simulink model "SF049A_LoaMgr"  (R2013b)
settings: Solver=FixedStepDiscrete  SolverMode=SingleTasking  StartTime=0.0  StopTime=1  FixedStep=0.002  RelTol=1e-3
values from neighbouring files (symbols this model uses):
  CURRMEASLOAMTGTNMASK_CNT_U08 = DataDict.Constant    [SF049A_LoaMgr_DataDict.m]
  IVTRLOAMTGTNMASK_CNT_U08 = DataDict.Constant    [SF049A_LoaMgr_DataDict.m]
  LOAMAXSLEW_ULSPERSEC_F32 = DataDict.Constant    [SF049A_LoaMgr_DataDict.m]
  LoaMgrCurrIvtrMtgtnRate = DataDict.Calibration    [SF049A_LoaMgr_DataDict.m]
  LoaMgrCurrIvtrMtgtnSca = DataDict.Calibration    [SF049A_LoaMgr_DataDict.m]
  LoaMgrCurrIvtrMtgtnScaZeroEna = DataDict.Calibration    [SF049A_LoaMgr_DataDict.m]
  LoaMgrCurrMeasIdptSig0Resp = DataDict.Calibration    [SF049A_LoaMgr_DataDict.m]
  LoaMgrCurrMeasIdptSig1Resp = DataDict.Calibration    [SF049A_LoaMgr_DataDict.m]
  LoaMgrCurrMeasIdptSig2Resp = DataDict.Calibration    [SF049A_LoaMgr_DataDict.m]
  LoaMgrCurrMeasIdptSigFltThd = DataDict.Calibration    [SF049A_LoaMgr_DataDict.m]
  LoaMgrCurrMeasMtgtnRate = DataDict.Calibration    [SF049A_LoaMgr_DataDict.m]
  LoaMgrCurrMeasMtgtnSca = DataDict.Calibration    [SF049A_LoaMgr_DataDict.m]
  LoaMgrCurrMeasMtgtnScaZeroEna = DataDict.Calibration    [SF049A_LoaMgr_DataDict.m]
  LoaMgrFadeOutStRate = DataDict.Calibration    [SF049A_LoaMgr_DataDict.m]
  LoaMgrHwTqIdptSig0NoTqLoaResp = DataDict.Calibration    [SF049A_LoaMgr_DataDict.m]
  LoaMgrHwTqIdptSig1NoTqLoaResp = DataDict.Calibration    [SF049A_LoaMgr_DataDict.m]
  LoaMgrHwTqIdptSig2Resp = DataDict.Calibration    [SF049A_LoaMgr_DataDict.m]
  LoaMgrHwTqIdptSig4Resp = DataDict.Calibration    [SF049A_LoaMgr_DataDict.m]
  LoaMgrHwTqIdptSigFltThd = DataDict.Calibration    [SF049A_LoaMgr_DataDict.m]
  LoaMgrHwTqLoaAvlResp = DataDict.Calibration    [SF049A_LoaMgr_DataDict.m]
  LoaMgrIvtrIdptSig0Resp = DataDict.Calibration    [SF049A_LoaMgr_DataDict.m]
  LoaMgrIvtrIdptSig1Resp = DataDict.Calibration    [SF049A_LoaMgr_DataDict.m]
  LoaMgrIvtrIdptSig2Resp = DataDict.Calibration    [SF049A_LoaMgr_DataDict.m]
  LoaMgrIvtrIdptSigFltThd = DataDict.Calibration    [SF049A_LoaMgr_DataDict.m]
  LoaMgrIvtrMtgtnRate = DataDict.Calibration    [SF049A_LoaMgr_DataDict.m]
  LoaMgrIvtrMtgtnSca = DataDict.Calibration    [SF049A_LoaMgr_DataDict.m]
  LoaMgrIvtrMtgtnScaZeroEna = DataDict.Calibration    [SF049A_LoaMgr_DataDict.m]
  LoaMgrLimdStRate = DataDict.Calibration    [SF049A_LoaMgr_DataDict.m]
  LoaMgrLimdStSca = DataDict.Calibration    [SF049A_LoaMgr_DataDict.m]
  LoaMgrMotAgAvlSnsrlsResp = DataDict.Calibration    [SF049A_LoaMgr_DataDict.m]
  LoaMgrMotAgIdptSig0NoSnsrlsResp = DataDict.Calibration    [SF049A_LoaMgr_DataDict.m]
  LoaMgrMotAgIdptSig1NoSnsrlsResp = DataDict.Calibration    [SF049A_LoaMgr_DataDict.m]
  LoaMgrMotAgIdptSig2Resp = DataDict.Calibration    [SF049A_LoaMgr_DataDict.m]
  LoaMgrMotAgIdptSig3Resp = DataDict.Calibration    [SF049A_LoaMgr_DataDict.m]
  LoaMgrMotAgIdptSigFltThd = DataDict.Calibration    [SF049A_LoaMgr_DataDict.m]
  LoaMgrMotAgMtgtnRate = DataDict.Calibration    [SF049A_LoaMgr_DataDict.m]
  LoaMgrMotAgMtgtnSca = DataDict.Calibration    [SF049A_LoaMgr_DataDict.m]
  LoaMgrMotAgMtgtnScaZeroEna = DataDict.Calibration    [SF049A_LoaMgr_DataDict.m]
  LOASCAONE_ULS_F32 = DataDict.Constant    [SF049A_LoaMgr_DataDict.m]
  LOASCAZERO_ULS_F32 = DataDict.Constant    [SF049A_LoaMgr_DataDict.m]
  LOASTIMDTSHTDWN_CNT_U08 = DataDict.Constant    [SF049A_LoaMgr_DataDict.m]
  LOASTNORM_CNT_U08 = DataDict.Constant    [SF049A_LoaMgr_DataDict.m]
  LOASTSWMTGTN_CNT_U08 = DataDict.Constant    [SF049A_LoaMgr_DataDict.m]
  MAXCURRMEASIDPTSIGALLWD_CNT_U08 = DataDict.Constant    [SF049A_LoaMgr_DataDict.m]
  MAXHWTQIDPTSIGALLWD_CNT_U08 = DataDict.Constant    [SF049A_LoaMgr_DataDict.m]
  MAXIVTRIDPTSIGALLWD_CNT_U08 = DataDict.Constant    [SF049A_LoaMgr_DataDict.m]
  MAXMOTAGMECLIDPTSIGALLWD_CNT_U08 = DataDict.Constant    [SF049A_LoaMgr_DataDict.m]
  NODEBSTEP_CNT_U16 = DataDict.Constant    [SF049A_LoaMgr_DataDict.m]
undefined symbols (not defined in the file or in its folder): LoaSt1, NtcNr1, NtcSts1, SigQlfr1
libraries: simulink x43, NxtrMin x4, NxtrMax x4, NxtrLim x2
(part 3 of 8)

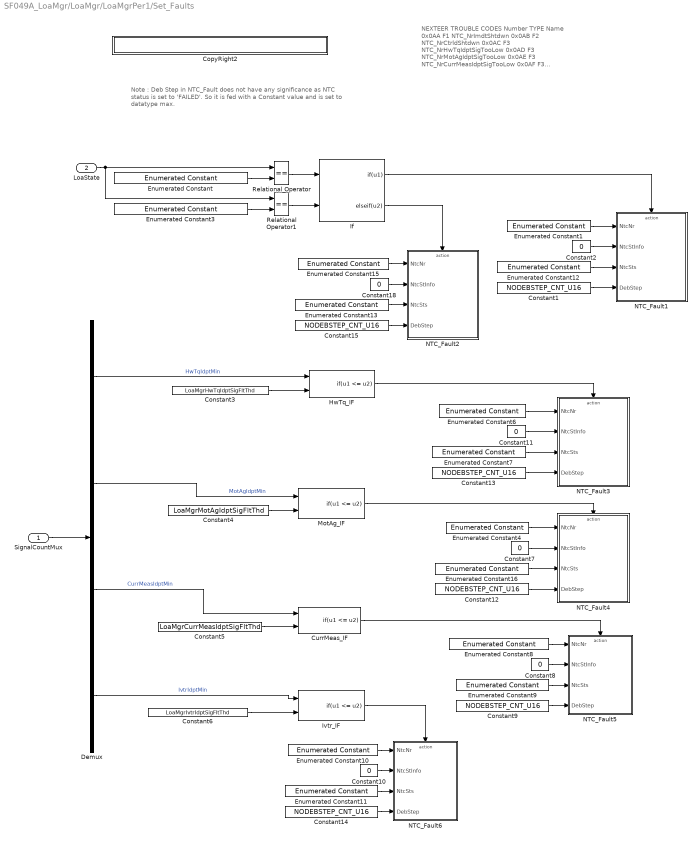
== system SF049A_LoaMgr/LoaMgr/LoaMgrPer1/Set_Faults ==
  note: Note : Deb Step in NTC_Fault does not have any significance as
      | NTC status is set to 'FAILED'. So it is fed with a Constant value and
      | is set to datatype max.
  note: NEXTEER TROUBLE CODES
      | Number  TYPE   Name
      |  0x0AA      F1      NTC_NrImdtShtdwn
      |  0x0AB      F2      NTC_NrCtrldShtdwn
      |  0x0AC      F3      NTC_NrHwTqIdptSigTooLow
      |  0x0AD      F3      NTC_NrMotAgIdptSigTooLow
      |  0x0AE      F3      NTC_NrCurrMeasIdptSigTooLow
      |  0x0AF      F3      NTC_NrIvtrIdptSigTooLow
  SignalCountMux : Inport
  LoaState : Inport  RequirementInfo="{'linktype_rmi_doors' '0000bab3 (/E-STEER Core/SubSystem Specifications/Application Functions/SF049A Loss of Assist Manager)' '#SF049A_115' 'true' 'REQ:  SF049A_115' '' ; 'linktype_rmi_doors' '0000bab3 (/E-STEER Core/SubSystem Specifications/Application Functions/SF049A Loss of Assist Manager)' '#SF049A_118' 'true' 'REQ:  SF049A_118' '' } %GIDa_4967d76f_74bb_495b_9f1d_be295f669af9"  Port=2
  Constant{1,9,12..15} (6 alike) : Constant  Value=NODEBSTEP_CNT_U16
  Constant{2,7..8,10..11,18} (6 alike) : Constant  Value=0
  Constant3 : Constant  RequirementInfo="{'linktype_rmi_doors' '0000bab3 (/E-STEER Core/SubSystem Specifications/Application Functions/SF049A Loss of Assist Manager)' '#SF049A_127' 'true' 'REQ:  SF049A_127' '' } %GIDa_3c5e0169_e7e2_4269_822a_0506f737a0d4"  Value=LoaMgrHwTqIdptSigFltThd  OutDataTypeStr=uint8
  Constant4 : Constant  RequirementInfo="{'linktype_rmi_doors' '0000bab3 (/E-STEER Core/SubSystem Specifications/Application Functions/SF049A Loss of Assist Manager)' '#SF049A_136' 'true' 'REQ:  SF049A_136' '' } %GIDa_abce65b2_de1a_4f6f_b7d5_5b7546b3af4d"  Value=LoaMgrMotAgIdptSigFltThd  OutDataTypeStr=uint8
  Constant5 : Constant  RequirementInfo="{'linktype_rmi_doors' '0000bab3 (/E-STEER Core/SubSystem Specifications/Application Functions/SF049A Loss of Assist Manager)' '#SF049A_145' 'true' 'REQ:  SF049A_145' '' } %GIDa_8ca978df_ec13_4868_a0a0_36ae85151f3c"  Value=LoaMgrCurrMeasIdptSigFltThd  OutDataTypeStr=uint8
  Constant6 : Constant  RequirementInfo="{'linktype_rmi_doors' '0000bab3 (/E-STEER Core/SubSystem Specifications/Application Functions/SF049A Loss of Assist Manager)' '#SF049A_154' 'true' 'REQ:  SF049A_154' '' } %GIDa_e4e38833_0b1e_42a6_94e4_589df1509d92"  Value=LoaMgrIvtrIdptSigFltThd  OutDataTypeStr=uint8
  CopyRight2 : Subsystem  Description=|  mask(Copyright Information){none=on}
      | Copyright info block.                                               
      |                                                                     
      | Place copyright information at the top of every subsystem in design.
      mask prompts: none "No parameters"
      mask help: Place copyright information at the top of every subsystem in design.
      mask Display:
      | NxtrConf = 'Nexteer Confidential';
      | 
      | sys = bdroot; %handle for the current model ("system")
      | first = get_param(sys,'Created');
      | first = first(end-3:end);  %year is last four digits
      | 
      | last = get_param(sys,'LastModifiedDate');
      | if isempty(last)
      |     last = datestr(now,'yyyy');
      | else
      |     last = last(end-3:end);
      | end
      | 
      | if strcmp(first,last)
      |     fprintf('%s -- Copyright %s Nexteer',NxtrConf,first)
      | else
      |     fprintf('%s -- %s%s- %s Nexteer',NxtrConf,char(169),first,last)
      | end
  CurrMeas_IF : If  RequirementInfo="{'linktype_rmi_doors' '0000bab3 (/E-STEER Core/SubSystem Specifications/Application Functions/SF049A Loss of Assist Manager)' '#SF049A_145' 'true' 'REQ:  SF049A_145' '' } %GIDa_23c69e12_f1ab_48c3_a465_95305b9e4132"  NumInputs=2  IfExpression=u1 <= u2  ShowElse=off
  Demux : Demux
  Enumerated Constant1 : simulink/Sources/Enumerated Constant  OutDataTypeStr=Enum: NtcNr1  Value=NtcNr1.NTCNR_0X0AA  SampleTime=inf
  Enumerated Constant10 : simulink/Sources/Enumerated Constant  OutDataTypeStr=Enum: NtcNr1  Value=NtcNr1.NTCNR_0X0AF  SampleTime=inf
  Enumerated Constant{7,9,11..13,16} (6 alike) : simulink/Sources/Enumerated Constant  OutDataTypeStr=Enum: NtcSts1  Value=NtcSts1.NTCSTS_FAILD  SampleTime=inf
  Enumerated Constant15 : simulink/Sources/Enumerated Constant  OutDataTypeStr=Enum: NtcNr1  Value=NtcNr1.NTCNR_0X0AB  SampleTime=inf
  Enumerated Constant4 : simulink/Sources/Enumerated Constant  OutDataTypeStr=Enum: NtcNr1  Value=NtcNr1.NTCNR_0X0AD  SampleTime=inf
  Enumerated Constant6 : simulink/Sources/Enumerated Constant  OutDataTypeStr=Enum: NtcNr1  Value=NtcNr1.NTCNR_0X0AC  SampleTime=inf
  Enumerated Constant8 : simulink/Sources/Enumerated Constant  OutDataTypeStr=Enum: NtcNr1  Value=NtcNr1.NTCNR_0X0AE  SampleTime=inf
  Enumerated Constant : simulink/Sources/Enumerated Constant  RequirementInfo="{'linktype_rmi_doors' '0000bab3 (/E-STEER Core/SubSystem Specifications/Application Functions/SF049A Loss of Assist Manager)' '#SF049A_115' 'true' 'REQ:  SF049A_115' '' } %GIDa_7720fc81_938d_420c_9ced_1233460611ba"  OutDataTypeStr=Enum: LoaSt1  Value=LoaSt1.LOAST_IMDTSHTDWNREQD  SampleTime=inf
  Enumerated Constant3 : simulink/Sources/Enumerated Constant  RequirementInfo="{'linktype_rmi_doors' '0000bab3 (/E-STEER Core/SubSystem Specifications/Application Functions/SF049A Loss of Assist Manager)' '#SF049A_118' 'true' 'REQ:  SF049A_118' '' } %GIDa_0b8c704e_8242_4dec_ad1d_b890924ca18f"  OutDataTypeStr=Enum: LoaSt1  Value=LoaSt1.LOAST_CTRLDSHTDWNREQD  SampleTime=inf
  HwTq_IF : If  RequirementInfo="{'linktype_rmi_doors' '0000bab3 (/E-STEER Core/SubSystem Specifications/Application Functions/SF049A Loss of Assist Manager)' '#SF049A_127' 'true' 'REQ:  SF049A_127' '' } %GIDa_c1a54aec_df59_476e_b8a2_fe90d0d01382"  NumInputs=2  IfExpression=u1 <= u2  ShowElse=off
  If : If  RequirementInfo="{'linktype_rmi_doors' '0000bab3 (/E-STEER Core/SubSystem Specifications/Application Functions/SF049A Loss of Assist Manager)' '#SF049A_115' 'true' 'REQ:  SF049A_115' '' ; 'linktype_rmi_doors' '0000bab3 (/E-STEER Core/SubSystem Specifications/Application Functions/SF049A Loss of Assist Manager)' '#SF049A_118' 'true' 'REQ:  SF049A_118' '' } %GIDa_2ae57359_ddcb_46c2_bc65_be72e5cb3771"  NumInputs=2  IfExpression=u1  ElseIfExpressions=u2  ShowElse=off
  Ivtr_IF : If  RequirementInfo="{'linktype_rmi_doors' '0000bab3 (/E-STEER Core/SubSystem Specifications/Application Functions/SF049A Loss of Assist Manager)' '#SF049A_154' 'true' 'REQ:  SF049A_154' '' } %GIDa_9e953e66_734a_4534_a97e_ce62b3d493b7"  NumInputs=2  IfExpression=u1 <= u2  ShowElse=off
  MotAg_IF : If  RequirementInfo="{'linktype_rmi_doors' '0000bab3 (/E-STEER Core/SubSystem Specifications/Application Functions/SF049A Loss of Assist Manager)' '#SF049A_136' 'true' 'REQ:  SF049A_136' '' } %GIDa_2fb2f3b7_b2e9_48d1_9bc3_88796399833b"  NumInputs=2  IfExpression=u1 <= u2  ShowElse=off
  NTC_Fault1 : Subsystem  mask(SetNTC){}
      mask help: SetNTC library block
  NTC_Fault2 : Subsystem  mask(SetNTC){}
      mask help: SetNTC library block
  NTC_Fault3 : Subsystem  mask(SetNTC){}
      mask help: SetNTC library block
  NTC_Fault4 : Subsystem  mask(SetNTC){}
      mask help: SetNTC library block
  NTC_Fault5 : Subsystem  mask(SetNTC){}
      mask help: SetNTC library block
  NTC_Fault6 : Subsystem  mask(SetNTC){}
      mask help: SetNTC library block
  Relational Operator : RelationalOperator  RequirementInfo="{'linktype_rmi_doors' '0000bab3 (/E-STEER Core/SubSystem Specifications/Application Functions/SF049A Loss of Assist Manager)' '#SF049A_115' 'true' 'REQ:  SF049A_115' '' } %GIDa_f05a48eb_4c6a_4aaa_9a59_9f6400fec108"  Operator===  OutDataTypeStr=boolean
  Relational Operator1 : RelationalOperator  RequirementInfo="{'linktype_rmi_doors' '0000bab3 (/E-STEER Core/SubSystem Specifications/Application Functions/SF049A Loss of Assist Manager)' '#SF049A_118' 'true' 'REQ:  SF049A_118' '' } %GIDa_4de44a16_c7b2_4a4a_90aa_5030e7b317ef"  Operator===  OutDataTypeStr=boolean
  wires:
  If/2 -> NTC_Fault2/Action
  If/1 -> NTC_Fault1/Action
  Enumerated Constant/1 -> Relational Operator/2
  Enumerated Constant3/1 -> Relational Operator1/2
  LoaState/1 -> Relational Operator/1, Relational Operator1/1
  Relational Operator1/1 -> If/2
  Relational Operator/1 -> If/1
  SignalCountMux/1 -> Demux/1
  Constant3/1 -> HwTq_IF/2
  Demux/1 -> HwTq_IF/1  "HwTqIdptMin"
  Constant4/1 -> MotAg_IF/2
  Demux/2 -> MotAg_IF/1  "MotAgIdptMin"
  Constant5/1 -> CurrMeas_IF/2
  Demux/3 -> CurrMeas_IF/1  "CurrMeasIdptMin"
  Constant6/1 -> Ivtr_IF/2
  Demux/4 -> Ivtr_IF/1  "IvtrIdptMin"
  HwTq_IF/1 -> NTC_Fault3/Action
  MotAg_IF/1 -> NTC_Fault4/Action
  Enumerated Constant8/1 -> NTC_Fault5/1(NtcNr)
  Constant8/1 -> NTC_Fault5/2(NtcStInfo)
  Enumerated Constant9/1 -> NTC_Fault5/3(NtcSts)
  Constant9/1 -> NTC_Fault5/4(DebStep)
  CurrMeas_IF/1 -> NTC_Fault5/Action
  Enumerated Constant10/1 -> NTC_Fault6/1(NtcNr)
  Constant10/1 -> NTC_Fault6/2(NtcStInfo)
  Enumerated Constant11/1 -> NTC_Fault6/3(NtcSts)
  Constant14/1 -> NTC_Fault6/4(DebStep)
  Ivtr_IF/1 -> NTC_Fault6/Action
  Constant15/1 -> NTC_Fault2/4(DebStep)
  Enumerated Constant13/1 -> NTC_Fault2/3(NtcSts)
  Constant18/1 -> NTC_Fault2/2(NtcStInfo)
  Enumerated Constant15/1 -> NTC_Fault2/1(NtcNr)
  Enumerated Constant1/1 -> NTC_Fault1/1(NtcNr)
  Constant2/1 -> NTC_Fault1/2(NtcStInfo)
  Enumerated Constant12/1 -> NTC_Fault1/3(NtcSts)
  Constant1/1 -> NTC_Fault1/4(DebStep)
  Enumerated Constant4/1 -> NTC_Fault4/1(NtcNr)
  Constant7/1 -> NTC_Fault4/2(NtcStInfo)
  Enumerated Constant16/1 -> NTC_Fault4/3(NtcSts)
  Constant12/1 -> NTC_Fault4/4(DebStep)
  Enumerated Constant6/1 -> NTC_Fault3/1(NtcNr)
  Constant11/1 -> NTC_Fault3/2(NtcStInfo)
  Enumerated Constant7/1 -> NTC_Fault3/3(NtcSts)
  Constant13/1 -> NTC_Fault3/4(DebStep)

== system SF049A_LoaMgr/LoaMgr/LoaMgrPer1/else ==
  In1 : Inport
  Action Port : ActionPort  ActionType=else
  Out1 : Outport
  wires:
  In1/1 -> Out1/1

== system SF049A_LoaMgr/LoaMgr/LoaMgrPer1/if ==
  Action Port : ActionPort  ActionType=then
  Constant : Constant  OutDataTypeStr=Inherit: Inherit via back propagation
  Out1 : Outport
  wires:
  Constant/1 -> Out1/1

== system SF049A_LoaMgr/ISO Fault Debounce/DiagMgr/NTCSTS_PREFAILD/CopyRight2 ==

== system SF049A_LoaMgr/ISO Fault Debounce/DiagMgr/NTCSTS_PREFAILD/If Action Subsystem ==
  DS : Inport
  Qlf : Inport  Port=2
  Action Port : ActionPort  ActionType=then
  EAo : Outport
  Qlfo : Outport  Port=2
  wires:
  Qlf/1 -> Qlfo/1
  DS/1 -> EAo/1

== system SF049A_LoaMgr/ISO Fault Debounce/DiagMgr/NTCSTS_PREFAILD/If Action Subsystem1 ==
  DS : Inport
  EA : Inport  Port=2
  Qlf : Inport  Port=3
  TS : Inport  Port=4
  Action Port : ActionPort  ActionType=else
  CopyRight2 : Subsystem  Description=|  mask(Copyright Information){none=on}
      | Copyright info block.                                               
      |                                                                     
      | Place copyright information at the top of every subsystem in design.
      mask prompts: none "No parameters"
      mask help: Place copyright information at the top of every subsystem in design.
      mask Display:
      | NxtrConf = 'Nexteer Confidential';
      | 
      | sys = bdroot; %handle for the current model ("system")
      | first = get_param(sys,'Created');
      | first = first(end-3:end);  %year is last four digits
      | 
      | last = get_param(sys,'LastModifiedDate');
      | if isempty(last)
      |     last = datestr(now,'yyyy');
      | else
      |     last = last(end-3:end);
      | end
      | 
      | if strcmp(first,last)
      |     fprintf('%s -- Copyright %s Nexteer',NxtrConf,first)
      | else
      |     fprintf('%s -- %s%s- %s Nexteer',NxtrConf,char(169),first,last)
      | end
  If : If  NumInputs=2  IfExpression=u1 < u2
  If Action Subsystem : Subsystem  TreatAsAtomicUnit=on
  If Action Subsystem1 : Subsystem  TreatAsAtomicUnit=on
  Merge : Merge
  Merge1 : Merge
  QFFailed : Constant  Value=SigQlfr1.SIGQLFR_FAILD  OutDataTypeStr=Enum: SigQlfr1
  Sum : Sum  Inputs=|++
  EAo : Outport
  Qlfo : Outport  Port=2
  wires:
  DS/1 -> Sum/1
  EA/1 -> Sum/2
  Sum/1 -> If Action Subsystem/1(EA), If/1
  TS/1 -> If Action Subsystem1/1(EA), If/2
  If/2 -> If Action Subsystem1/Action
  If/1 -> If Action Subsystem/Action
  Qlf/1 -> If Action Subsystem/2(Qlf)
  QFFailed/1 -> If Action Subsystem1/2(Qlf)
  Merge1/1 -> Qlfo/1
  Merge/1 -> EAo/1
  If Action Subsystem1/1(EAo) -> Merge/1
  If Action Subsystem/1(EAo) -> Merge/2
  If Action Subsystem1/2(Qlfo) -> Merge1/1
  If Action Subsystem/2(Qlfo) -> Merge1/2

== system SF049A_LoaMgr/ISO Fault Debounce/DiagMgr/NTCSTS_PREPASSD/CopyRight2 ==

== system SF049A_LoaMgr/ISO Fault Debounce/DiagMgr/NTCSTS_PREPASSD/If Action Subsystem ==
  In1 : Inport
  In2 : Inport  Port=2
  Action Port : ActionPort  ActionType=then
  Out1 : Outport
  Out2 : Outport  Port=2
  wires:
  In1/1 -> Out1/1
  In2/1 -> Out2/1

== system SF049A_LoaMgr/ISO Fault Debounce/DiagMgr/NTCSTS_PREPASSD/If Action Subsystem1 ==
  In1 : Inport
  In2 : Inport  Port=2
  Action Port : ActionPort  ActionType=else
  Out1 : Outport
  Out2 : Outport  Port=2
  wires:
  In1/1 -> Out1/1
  In2/1 -> Out2/1

== system SF049A_LoaMgr/LoaMgr/LoaMgrInit1/NTC_Fault1/SetNtcSts ==
  NtcNr : Inport
  NtcStInfo : Inport  Port=2
  NtcSts : Inport  Port=3
  DebStep : Inport  Port=4
  CopyRight2 : Subsystem  Description=|  mask(Copyright Information){none=on}
      | Copyright info block.                                               
      |                                                                     
      | Place copyright information at the top of every subsystem in design.
      mask prompts: none "No parameters"
      mask help: Place copyright information at the top of every subsystem in design.
      mask Display:
      | NxtrConf = 'Nexteer Confidential';
      | 
      | sys = bdroot; %handle for the current model ("system")
      | first = get_param(sys,'Created');
      | first = first(end-3:end);  %year is last four digits
      | 
      | last = get_param(sys,'LastModifiedDate');
      | if isempty(last)
      |     last = datestr(now,'yyyy');
      | else
      |     last = last(end-3:end);
      | end
      | 
      | if strcmp(first,last)
      |     fprintf('%s -- Copyright %s Nexteer',NxtrConf,first)
      | else
      |     fprintf('%s -- %s%s- %s Nexteer',NxtrConf,char(169),first,last)
      | end
  Data Store Write1 : DataStoreWrite  DataStoreName=DebStep
  Data Store Write3 : DataStoreWrite  DataStoreName=Fault1_Status
  Terminator : Terminator
  Terminator1 : Terminator
  wires:
  NtcStInfo/1 -> Terminator1/1
  NtcNr/1 -> Terminator/1
  NtcSts/1 -> Data Store Write3/1
  DebStep/1 -> Data Store Write1/1

== system SF049A_LoaMgr/LoaMgr/LoaMgrInit1/NTC_Fault2/SetNtcSts ==
  NtcNr : Inport
  NtcStInfo : Inport  Port=2
  NtcSts : Inport  Port=3
  DebStep : Inport  Port=4
  CopyRight2 : Subsystem  Description=|  mask(Copyright Information){none=on}
      | Copyright info block.                                               
      |                                                                     
      | Place copyright information at the top of every subsystem in design.
      mask prompts: none "No parameters"
      mask help: Place copyright information at the top of every subsystem in design.
      mask Display:
      | NxtrConf = 'Nexteer Confidential';
      | 
      | sys = bdroot; %handle for the current model ("system")
      | first = get_param(sys,'Created');
      | first = first(end-3:end);  %year is last four digits
      | 
      | last = get_param(sys,'LastModifiedDate');
      | if isempty(last)
      |     last = datestr(now,'yyyy');
      | else
      |     last = last(end-3:end);
      | end
      | 
      | if strcmp(first,last)
      |     fprintf('%s -- Copyright %s Nexteer',NxtrConf,first)
      | else
      |     fprintf('%s -- %s%s- %s Nexteer',NxtrConf,char(169),first,last)
      | end
  Data Store Write1 : DataStoreWrite  DataStoreName=DebStep
  Data Store Write3 : DataStoreWrite  DataStoreName=Fault2_Status
  Terminator : Terminator
  Terminator1 : Terminator
  wires:
  DebStep/1 -> Data Store Write1/1
  NtcSts/1 -> Data Store Write3/1
  NtcNr/1 -> Terminator/1
  NtcStInfo/1 -> Terminator1/1

== system SF049A_LoaMgr/LoaMgr/LoaMgrInit1/NTC_Fault3/SetNtcSts ==
  NtcNr : Inport
  NtcStInfo : Inport  Port=2
  NtcSts : Inport  Port=3
  DebStep : Inport  Port=4
  CopyRight2 : Subsystem  Description=|  mask(Copyright Information){none=on}
      | Copyright info block.                                               
      |                                                                     
      | Place copyright information at the top of every subsystem in design.
      mask prompts: none "No parameters"
      mask help: Place copyright information at the top of every subsystem in design.
      mask Display:
      | NxtrConf = 'Nexteer Confidential';
      | 
      | sys = bdroot; %handle for the current model ("system")
      | first = get_param(sys,'Created');
      | first = first(end-3:end);  %year is last four digits
      | 
      | last = get_param(sys,'LastModifiedDate');
      | if isempty(last)
      |     last = datestr(now,'yyyy');
      | else
      |     last = last(end-3:end);
      | end
      | 
      | if strcmp(first,last)
      |     fprintf('%s -- Copyright %s Nexteer',NxtrConf,first)
      | else
      |     fprintf('%s -- %s%s- %s Nexteer',NxtrConf,char(169),first,last)
      | end
  Data Store Write1 : DataStoreWrite  DataStoreName=DebStep
  Data Store Write3 : DataStoreWrite  DataStoreName=Fault3_Status
  Terminator : Terminator
  Terminator1 : Terminator
  wires:
  DebStep/1 -> Data Store Write1/1
  NtcSts/1 -> Data Store Write3/1
  NtcNr/1 -> Terminator/1
  NtcStInfo/1 -> Terminator1/1

== system SF049A_LoaMgr/LoaMgr/LoaMgrInit1/NTC_Fault4/SetNtcSts ==
  NtcNr : Inport
  NtcStInfo : Inport  Port=2
  NtcSts : Inport  Port=3
  DebStep : Inport  Port=4
  CopyRight2 : Subsystem  Description=|  mask(Copyright Information){none=on}
      | Copyright info block.                                               
      |                                                                     
      | Place copyright information at the top of every subsystem in design.
      mask prompts: none "No parameters"
      mask help: Place copyright information at the top of every subsystem in design.
      mask Display:
      | NxtrConf = 'Nexteer Confidential';
      | 
      | sys = bdroot; %handle for the current model ("system")
      | first = get_param(sys,'Created');
      | first = first(end-3:end);  %year is last four digits
      | 
      | last = get_param(sys,'LastModifiedDate');
      | if isempty(last)
      |     last = datestr(now,'yyyy');
      | else
      |     last = last(end-3:end);
      | end
      | 
      | if strcmp(first,last)
      |     fprintf('%s -- Copyright %s Nexteer',NxtrConf,first)
      | else
      |     fprintf('%s -- %s%s- %s Nexteer',NxtrConf,char(169),first,last)
      | end
  Data Store Write1 : DataStoreWrite  DataStoreName=DebStep
  Data Store Write3 : DataStoreWrite  DataStoreName=Fault4_Status
  Terminator : Terminator
  Terminator1 : Terminator
  wires:
  NtcStInfo/1 -> Terminator1/1
  NtcNr/1 -> Terminator/1
  NtcSts/1 -> Data Store Write3/1
  DebStep/1 -> Data Store Write1/1

== system SF049A_LoaMgr/LoaMgr/LoaMgrInit1/NTC_Fault5/SetNtcSts ==
  NtcNr : Inport
  NtcStInfo : Inport  Port=2
  NtcSts : Inport  Port=3
  DebStep : Inport  Port=4
  CopyRight2 : Subsystem  Description=|  mask(Copyright Information){none=on}
      | Copyright info block.                                               
      |                                                                     
      | Place copyright information at the top of every subsystem in design.
      mask prompts: none "No parameters"
      mask help: Place copyright information at the top of every subsystem in design.
      mask Display:
      | NxtrConf = 'Nexteer Confidential';
      | 
      | sys = bdroot; %handle for the current model ("system")
      | first = get_param(sys,'Created');
      | first = first(end-3:end);  %year is last four digits
      | 
      | last = get_param(sys,'LastModifiedDate');
      | if isempty(last)
      |     last = datestr(now,'yyyy');
      | else
      |     last = last(end-3:end);
      | end
      | 
      | if strcmp(first,last)
      |     fprintf('%s -- Copyright %s Nexteer',NxtrConf,first)
      | else
      |     fprintf('%s -- %s%s- %s Nexteer',NxtrConf,char(169),first,last)
      | end
  Data Store Write1 : DataStoreWrite  DataStoreName=DebStep
  Data Store Write3 : DataStoreWrite  DataStoreName=Fault5_Status
  Terminator : Terminator
  Terminator1 : Terminator
  wires:
  DebStep/1 -> Data Store Write1/1
  NtcSts/1 -> Data Store Write3/1
  NtcNr/1 -> Terminator/1
  NtcStInfo/1 -> Terminator1/1

== system SF049A_LoaMgr/LoaMgr/LoaMgrInit1/NTC_Fault6/SetNtcSts ==
  NtcNr : Inport
  NtcStInfo : Inport  Port=2
  NtcSts : Inport  Port=3
  DebStep : Inport  Port=4
  CopyRight2 : Subsystem  Description=|  mask(Copyright Information){none=on}
      | Copyright info block.                                               
      |                                                                     
      | Place copyright information at the top of every subsystem in design.
      mask prompts: none "No parameters"
      mask help: Place copyright information at the top of every subsystem in design.
      mask Display:
      | NxtrConf = 'Nexteer Confidential';
      | 
      | sys = bdroot; %handle for the current model ("system")
      | first = get_param(sys,'Created');
      | first = first(end-3:end);  %year is last four digits
      | 
      | last = get_param(sys,'LastModifiedDate');
      | if isempty(last)
      |     last = datestr(now,'yyyy');
      | else
      |     last = last(end-3:end);
      | end
      | 
      | if strcmp(first,last)
      |     fprintf('%s -- Copyright %s Nexteer',NxtrConf,first)
      | else
      |     fprintf('%s -- %s%s- %s Nexteer',NxtrConf,char(169),first,last)
      | end
  Data Store Write1 : DataStoreWrite  DataStoreName=DebStep
  Data Store Write3 : DataStoreWrite  DataStoreName=Fault6_Status
  Terminator : Terminator
  Terminator1 : Terminator
  wires:
  DebStep/1 -> Data Store Write1/1
  NtcSts/1 -> Data Store Write3/1
  NtcNr/1 -> Terminator/1
  NtcStInfo/1 -> Terminator1/1

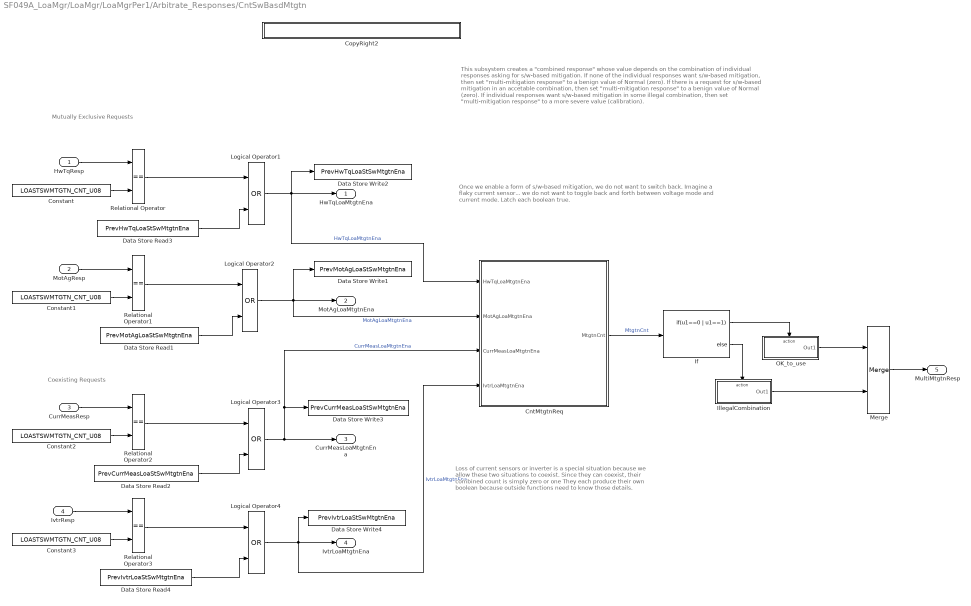
== system SF049A_LoaMgr/LoaMgr/LoaMgrPer1/Arbitrate_Responses/CntSwBasdMtgtn ==
  note: Coexisting Requests
  note: Mutually Exclusive Requests
  note: This subsystem creates a "combined response" whose value depends on the combination of individual responses asking for s/w-based mitigation.
      |    If none of the individual responses want s/w-based mitigation,                          then set "multi-mitigation response" to a benign value of Normal (zero).
      |    If there is a request for s/w-based mitigation in an accetable combination,        then set "multi-mitigation response" to a benign value of Normal (zero).
      |    If individual responses want s/w-based mitigation in some illegal combination, then set "multi-mitigation response" to a more severe value (calibration).
  note: Once we enable a form of s/w-based mitigation, we do not want to switch back.  Imagine
      | a flaky current sensor... we do not want to toggle back and forth between voltage mode
      | and current mode.  Latch each boolean true.
  note: Loss of current sensors or inverter is a special situation because
      | we allow these two situations to coexist.  Since they can coexist,
      | their combined count is simply zero or one
      |
      | They each produce their own boolean because outside functions
      | need to know those details.
  HwTqResp : Inport  RequirementInfo="{'linktype_rmi_doors' '0000bab3 (/E-STEER Core/SubSystem Specifications/Application Functions/SF049A Loss of Assist Manager)' '#SF049A_68' 'true' 'REQ:  SF049A_68' '' ; 'linktype_rmi_doors' '0000bab3 (/E-STEER Core/SubSystem Specifications/Application Functions/SF049A Loss of Assist Manager)' '#SF049A_69' 'true' 'REQ:  SF049A_69' '' } %GIDa_b80d0f50_f90b_4e03_8466_83f2cf72d7d0"
  MotAgResp : Inport  RequirementInfo="{'linktype_rmi_doors' '0000bab3 (/E-STEER Core/SubSystem Specifications/Application Functions/SF049A Loss of Assist Manager)' '#SF049A_70' 'true' 'REQ:  SF049A_70' '' ; 'linktype_rmi_doors' '0000bab3 (/E-STEER Core/SubSystem Specifications/Application Functions/SF049A Loss of Assist Manager)' '#SF049A_71' 'true' 'REQ:  SF049A_71' '' } %GIDa_2494d399_79f4_430f_9f1c_729d22ef6b78"  Port=2
  CurrMeasResp : Inport  RequirementInfo="{'linktype_rmi_doors' '0000bab3 (/E-STEER Core/SubSystem Specifications/Application Functions/SF049A Loss of Assist Manager)' '#SF049A_72' 'true' 'REQ:  SF049A_72' '' ; 'linktype_rmi_doors' '0000bab3 (/E-STEER Core/SubSystem Specifications/Application Functions/SF049A Loss of Assist Manager)' '#SF049A_73' 'true' 'REQ:  SF049A_73' '' } %GIDa_f0510da4_ee85_44f3_ba01_49a17aedb234"  Port=3
  IvtrResp : Inport  RequirementInfo="{'linktype_rmi_doors' '0000bab3 (/E-STEER Core/SubSystem Specifications/Application Functions/SF049A Loss of Assist Manager)' '#SF049A_74' 'true' 'REQ:  SF049A_74' '' ; 'linktype_rmi_doors' '0000bab3 (/E-STEER Core/SubSystem Specifications/Application Functions/SF049A Loss of Assist Manager)' '#SF049A_75' 'true' 'REQ:  SF049A_75' '' } %GIDa_c794d8ae_615d_487c_a87b_47bad332765b"  Port=4
  CntMtgtnReq : Subsystem
  Constant : Constant  RequirementInfo="{'linktype_rmi_doors' '0000bab3 (/E-STEER Core/SubSystem Specifications/Application Functions/SF049A Loss of Assist Manager)' '#SF049A_68' 'true' 'REQ:  SF049A_68' '' ; 'linktype_rmi_doors' '0000bab3 (/E-STEER Core/SubSystem Specifications/Application Functions/SF049A Loss of Assist Manager)' '#SF049A_69' 'true' 'REQ:  SF049A_69' '' } %GIDa_bd9a3dd1_2e5d_4476_962e_6318fd5d1be8"  Value=LOASTSWMTGTN_CNT_U08
  Constant1 : Constant  RequirementInfo="{'linktype_rmi_doors' '0000bab3 (/E-STEER Core/SubSystem Specifications/Application Functions/SF049A Loss of Assist Manager)' '#SF049A_70' 'true' 'REQ:  SF049A_70' '' ; 'linktype_rmi_doors' '0000bab3 (/E-STEER Core/SubSystem Specifications/Application Functions/SF049A Loss of Assist Manager)' '#SF049A_71' 'true' 'REQ:  SF049A_71' '' } %GIDa_dfd0b419_17dc_43f3_ad41_648a5721e57f"  Value=LOASTSWMTGTN_CNT_U08
  Constant2 : Constant  RequirementInfo="{'linktype_rmi_doors' '0000bab3 (/E-STEER Core/SubSystem Specifications/Application Functions/SF049A Loss of Assist Manager)' '#SF049A_72' 'true' 'REQ:  SF049A_72' '' ; 'linktype_rmi_doors' '0000bab3 (/E-STEER Core/SubSystem Specifications/Application Functions/SF049A Loss of Assist Manager)' '#SF049A_73' 'true' 'REQ:  SF049A_73' '' } %GIDa_2838f02e_7ff5_4ce5_9c2c_8ac453577de9"  Value=LOASTSWMTGTN_CNT_U08
  Constant3 : Constant  RequirementInfo="{'linktype_rmi_doors' '0000bab3 (/E-STEER Core/SubSystem Specifications/Application Functions/SF049A Loss of Assist Manager)' '#SF049A_74' 'true' 'REQ:  SF049A_74' '' ; 'linktype_rmi_doors' '0000bab3 (/E-STEER Core/SubSystem Specifications/Application Functions/SF049A Loss of Assist Manager)' '#SF049A_75' 'true' 'REQ:  SF049A_75' '' } %GIDa_e6d6bdaa_3e25_40eb_a3d0_c599cce94c1e"  Value=LOASTSWMTGTN_CNT_U08
  CopyRight2 : Subsystem  Description=|  mask(Copyright Information){none=on}
      | Copyright info block.                                               
      |                                                                     
      | Place copyright information at the top of every subsystem in design.
      mask prompts: none "No parameters"
      mask help: Place copyright information at the top of every subsystem in design.
      mask Display:
      | NxtrConf = 'Nexteer Confidential';
      | 
      | sys = bdroot; %handle for the current model ("system")
      | first = get_param(sys,'Created');
      | first = first(end-3:end);  %year is last four digits
      | 
      | last = get_param(sys,'LastModifiedDate');
      | if isempty(last)
      |     last = datestr(now,'yyyy');
      | else
      |     last = last(end-3:end);
      | end
      | 
      | if strcmp(first,last)
      |     fprintf('%s -- Copyright %s Nexteer',NxtrConf,first)
      | else
      |     fprintf('%s -- %s%s- %s Nexteer',NxtrConf,char(169),first,last)
      | end
  Data Store Read1 : DataStoreRead  RequirementInfo="{'linktype_rmi_doors' '0000bab3 (/E-STEER Core/SubSystem Specifications/Application Functions/SF049A Loss of Assist Manager)' '#SF049A_70' 'true' 'REQ:  SF049A_70' '' ; 'linktype_rmi_doors' '0000bab3 (/E-STEER Core/SubSystem Specifications/Application Functions/SF049A Loss of Assist Manager)' '#SF049A_71' 'true' 'REQ:  SF049A_71' '' } %GIDa_3b3697c5_1c5e_41ed_b14e_fe5ec1808ddf"  DataStoreName=PrevMotAgLoaStSwMtgtnEna
  Data Store Read2 : DataStoreRead  RequirementInfo="{'linktype_rmi_doors' '0000bab3 (/E-STEER Core/SubSystem Specifications/Application Functions/SF049A Loss of Assist Manager)' '#SF049A_72' 'true' 'REQ:  SF049A_72' '' ; 'linktype_rmi_doors' '0000bab3 (/E-STEER Core/SubSystem Specifications/Application Functions/SF049A Loss of Assist Manager)' '#SF049A_73' 'true' 'REQ:  SF049A_73' '' } %GIDa_c5d6354c_cd68_442f_9ee5_716caeef47d3"  DataStoreName=PrevCurrMeasLoaStSwMtgtnEna
  Data Store Read3 : DataStoreRead  RequirementInfo="{'linktype_rmi_doors' '0000bab3 (/E-STEER Core/SubSystem Specifications/Application Functions/SF049A Loss of Assist Manager)' '#SF049A_68' 'true' 'REQ:  SF049A_68' '' ; 'linktype_rmi_doors' '0000bab3 (/E-STEER Core/SubSystem Specifications/Application Functions/SF049A Loss of Assist Manager)' '#SF049A_69' 'true' 'REQ:  SF049A_69' '' } %GIDa_37a54a63_cd92_485a_b58e_f7c55d1647b3"  DataStoreName=PrevHwTqLoaStSwMtgtnEna
  Data Store Read4 : DataStoreRead  RequirementInfo="{'linktype_rmi_doors' '0000bab3 (/E-STEER Core/SubSystem Specifications/Application Functions/SF049A Loss of Assist Manager)' '#SF049A_74' 'true' 'REQ:  SF049A_74' '' ; 'linktype_rmi_doors' '0000bab3 (/E-STEER Core/SubSystem Specifications/Application Functions/SF049A Loss of Assist Manager)' '#SF049A_75' 'true' 'REQ:  SF049A_75' '' } %GIDa_3b2a642d_9a93_4cf9_8bb0_ebe0ce9c740b"  DataStoreName=PrevIvtrLoaStSwMtgtnEna
  Data Store Write1 : DataStoreWrite  RequirementInfo="{'linktype_rmi_doors' '0000bab3 (/E-STEER Core/SubSystem Specifications/Application Functions/SF049A Loss of Assist Manager)' '#SF049A_70' 'true' 'REQ:  SF049A_70' '' ; 'linktype_rmi_doors' '0000bab3 (/E-STEER Core/SubSystem Specifications/Application Functions/SF049A Loss of Assist Manager)' '#SF049A_71' 'true' 'REQ:  SF049A_71' '' } %GIDa_e12ef025_4146_4f66_8165_3f8c10ffb94e"  DataStoreName=PrevMotAgLoaStSwMtgtnEna
  Data Store Write2 : DataStoreWrite  RequirementInfo="{'linktype_rmi_doors' '0000bab3 (/E-STEER Core/SubSystem Specifications/Application Functions/SF049A Loss of Assist Manager)' '#SF049A_68' 'true' 'REQ:  SF049A_68' '' ; 'linktype_rmi_doors' '0000bab3 (/E-STEER Core/SubSystem Specifications/Application Functions/SF049A Loss of Assist Manager)' '#SF049A_69' 'true' 'REQ:  SF049A_69' '' } %GIDa_47c6e733_ed31_40d1_ab25_dd6621fdd7fc"  DataStoreName=PrevHwTqLoaStSwMtgtnEna
  Data Store Write3 : DataStoreWrite  RequirementInfo="{'linktype_rmi_doors' '0000bab3 (/E-STEER Core/SubSystem Specifications/Application Functions/SF049A Loss of Assist Manager)' '#SF049A_72' 'true' 'REQ:  SF049A_72' '' ; 'linktype_rmi_doors' '0000bab3 (/E-STEER Core/SubSystem Specifications/Application Functions/SF049A Loss of Assist Manager)' '#SF049A_73' 'true' 'REQ:  SF049A_73' '' } %GIDa_79d53804_14a5_4666_9a8f_f334b27c0e19"  DataStoreName=PrevCurrMeasLoaStSwMtgtnEna
  Data Store Write4 : DataStoreWrite  RequirementInfo="{'linktype_rmi_doors' '0000bab3 (/E-STEER Core/SubSystem Specifications/Application Functions/SF049A Loss of Assist Manager)' '#SF049A_74' 'true' 'REQ:  SF049A_74' '' ; 'linktype_rmi_doors' '0000bab3 (/E-STEER Core/SubSystem Specifications/Application Functions/SF049A Loss of Assist Manager)' '#SF049A_75' 'true' 'REQ:  SF049A_75' '' } %GIDa_36c36165_4224_4644_b812_bf09f46fc7a3"  DataStoreName=PrevIvtrLoaStSwMtgtnEna
  If : If  RequirementInfo="{'linktype_rmi_doors' '0000bab3 (/E-STEER Core/SubSystem Specifications/Application Functions/SF049A Loss of Assist Manager)' '#SF049A_80' 'true' 'REQ:  SF049A_80' '' ; 'linktype_rmi_doors' '0000bab3 (/E-STEER Core/SubSystem Specifications/Application Functions/SF049A Loss of Assist Manager)' '#SF049A_81' 'true' 'REQ:  SF049A_81' '' ; 'linktype_rmi_doors' '0000bab3 (/E-STEER Core/SubSystem Specifications/Application Functions/SF049A Loss of Assist Manager)' '#SF049A_83' 'true' 'REQ:  SF049A_83' '' } %GIDa_66e0b8e0_46fd_4ab7_b007_3cd8f27f40de"  IfExpression=u1==0 | u1==1
  IllegalCombination : Subsystem  RequirementInfo="{'linktype_rmi_doors' '0000bab3 (/E-STEER Core/SubSystem Specifications/Application Functions/SF049A Loss of Assist Manager)' '#SF049A_80' 'true' 'REQ:  SF049A_80' '' ; 'linktype_rmi_doors' '0000bab3 (/E-STEER Core/SubSystem Specifications/Application Functions/SF049A Loss of Assist Manager)' '#SF049A_81' 'true' 'REQ:  SF049A_81' '' } %GIDa_b8b68a31_4a60_45e0_b898_416fd75d7a54"  TreatAsAtomicUnit=on
  Logical Operator1 : Logic  RequirementInfo="{'linktype_rmi_doors' '0000bab3 (/E-STEER Core/SubSystem Specifications/Application Functions/SF049A Loss of Assist Manager)' '#SF049A_68' 'true' 'REQ:  SF049A_68' '' ; 'linktype_rmi_doors' '0000bab3 (/E-STEER Core/SubSystem Specifications/Application Functions/SF049A Loss of Assist Manager)' '#SF049A_69' 'true' 'REQ:  SF049A_69' '' } %GIDa_b5ddf1d6_f654_4565_99aa_236dfe43585d"  Operator=OR  AllPortsSameDT=off  OutDataTypeStr=boolean
  Logical Operator2 : Logic  RequirementInfo="{'linktype_rmi_doors' '0000bab3 (/E-STEER Core/SubSystem Specifications/Application Functions/SF049A Loss of Assist Manager)' '#SF049A_70' 'true' 'REQ:  SF049A_70' '' ; 'linktype_rmi_doors' '0000bab3 (/E-STEER Core/SubSystem Specifications/Application Functions/SF049A Loss of Assist Manager)' '#SF049A_71' 'true' 'REQ:  SF049A_71' '' } %GIDa_19cbaa5c_3a0b_47ba_9315_98fd0668e5f9"  Operator=OR  AllPortsSameDT=off  OutDataTypeStr=boolean
  Logical Operator3 : Logic  RequirementInfo="{'linktype_rmi_doors' '0000bab3 (/E-STEER Core/SubSystem Specifications/Application Functions/SF049A Loss of Assist Manager)' '#SF049A_72' 'true' 'REQ:  SF049A_72' '' ; 'linktype_rmi_doors' '0000bab3 (/E-STEER Core/SubSystem Specifications/Application Functions/SF049A Loss of Assist Manager)' '#SF049A_73' 'true' 'REQ:  SF049A_73' '' } %GIDa_3e1ab1ab_6f26_4517_9fd4_d59b9b6d576b"  Operator=OR  AllPortsSameDT=off  OutDataTypeStr=boolean
  Logical Operator4 : Logic  RequirementInfo="{'linktype_rmi_doors' '0000bab3 (/E-STEER Core/SubSystem Specifications/Application Functions/SF049A Loss of Assist Manager)' '#SF049A_74' 'true' 'REQ:  SF049A_74' '' ; 'linktype_rmi_doors' '0000bab3 (/E-STEER Core/SubSystem Specifications/Application Functions/SF049A Loss of Assist Manager)' '#SF049A_75' 'true' 'REQ:  SF049A_75' '' } %GIDa_afc7672b_39c0_4c55_907f_4f5cfaa6621d"  Operator=OR  AllPortsSameDT=off  OutDataTypeStr=boolean
  Merge : Merge  RequirementInfo="{'linktype_rmi_doors' '0000bab3 (/E-STEER Core/SubSystem Specifications/Application Functions/SF049A Loss of Assist Manager)' '#SF049A_80' 'true' 'REQ:  SF049A_80' '' ; 'linktype_rmi_doors' '0000bab3 (/E-STEER Core/SubSystem Specifications/Application Functions/SF049A Loss of Assist Manager)' '#SF049A_81' 'true' 'REQ:  SF049A_81' '' ; 'linktype_rmi_doors' '0000bab3 (/E-STEER Core/SubSystem Specifications/Application Functions/SF049A Loss of Assist Manager)' '#SF049A_83' 'true' 'REQ:  SF049A_83' '' } %GIDa_4a2d78c3_4c4a_4f1b_85f7_0e10b037d212"
  OK_to_use : Subsystem  RequirementInfo="{'linktype_rmi_doors' '0000bab3 (/E-STEER Core/SubSystem Specifications/Application Functions/SF049A Loss of Assist Manager)' '#SF049A_80' 'true' 'REQ:  SF049A_80' '' ; 'linktype_rmi_doors' '0000bab3 (/E-STEER Core/SubSystem Specifications/Application Functions/SF049A Loss of Assist Manager)' '#SF049A_81' 'true' 'REQ:  SF049A_81' '' } %GIDa_b3cbff71_477b_4868_99de_c9cfcf1d411c"  TreatAsAtomicUnit=on
  Relational Operator : RelationalOperator  RequirementInfo="{'linktype_rmi_doors' '0000bab3 (/E-STEER Core/SubSystem Specifications/Application Functions/SF049A Loss of Assist Manager)' '#SF049A_68' 'true' 'REQ:  SF049A_68' '' ; 'linktype_rmi_doors' '0000bab3 (/E-STEER Core/SubSystem Specifications/Application Functions/SF049A Loss of Assist Manager)' '#SF049A_69' 'true' 'REQ:  SF049A_69' '' } %GIDa_a15a64f3_7000_43e4_9aa1_ad5ebae10911"  Operator===  OutDataTypeStr=boolean
  Relational Operator1 : RelationalOperator  RequirementInfo="{'linktype_rmi_doors' '0000bab3 (/E-STEER Core/SubSystem Specifications/Application Functions/SF049A Loss of Assist Manager)' '#SF049A_70' 'true' 'REQ:  SF049A_70' '' ; 'linktype_rmi_doors' '0000bab3 (/E-STEER Core/SubSystem Specifications/Application Functions/SF049A Loss of Assist Manager)' '#SF049A_71' 'true' 'REQ:  SF049A_71' '' } %GIDa_b00f9d20_7939_4e3e_85d4_0246b232e92d"  Operator===  OutDataTypeStr=boolean
  Relational Operator2 : RelationalOperator  RequirementInfo="{'linktype_rmi_doors' '0000bab3 (/E-STEER Core/SubSystem Specifications/Application Functions/SF049A Loss of Assist Manager)' '#SF049A_72' 'true' 'REQ:  SF049A_72' '' ; 'linktype_rmi_doors' '0000bab3 (/E-STEER Core/SubSystem Specifications/Application Functions/SF049A Loss of Assist Manager)' '#SF049A_73' 'true' 'REQ:  SF049A_73' '' } %GIDa_1b0ee92b_8a3f_4274_82fb_cab1558310dd"  Operator===  OutDataTypeStr=boolean
  Relational Operator3 : RelationalOperator  RequirementInfo="{'linktype_rmi_doors' '0000bab3 (/E-STEER Core/SubSystem Specifications/Application Functions/SF049A Loss of Assist Manager)' '#SF049A_74' 'true' 'REQ:  SF049A_74' '' ; 'linktype_rmi_doors' '0000bab3 (/E-STEER Core/SubSystem Specifications/Application Functions/SF049A Loss of Assist Manager)' '#SF049A_75' 'true' 'REQ:  SF049A_75' '' } %GIDa_da48cf5a_e7f7_492a_b79d_b1bb29b0e53d"  Operator===  OutDataTypeStr=boolean
  HwTqLoaMtgtnEna : Outport  RequirementInfo="{'linktype_rmi_doors' '0000bab3 (/E-STEER Core/SubSystem Specifications/Application Functions/SF049A Loss of Assist Manager)' '#SF049A_68' 'true' 'REQ:  SF049A_68' '' ; 'linktype_rmi_doors' '0000bab3 (/E-STEER Core/SubSystem Specifications/Application Functions/SF049A Loss of Assist Manager)' '#SF049A_69' 'true' 'REQ:  SF049A_69' '' } %GIDa_b6ff4eda_59b3_41e5_b66c_5ffa2aa858f3"
  MotAgLoaMtgtnEna : Outport  RequirementInfo="{'linktype_rmi_doors' '0000bab3 (/E-STEER Core/SubSystem Specifications/Application Functions/SF049A Loss of Assist Manager)' '#SF049A_70' 'true' 'REQ:  SF049A_70' '' ; 'linktype_rmi_doors' '0000bab3 (/E-STEER Core/SubSystem Specifications/Application Functions/SF049A Loss of Assist Manager)' '#SF049A_71' 'true' 'REQ:  SF049A_71' '' } %GIDa_1e1e14d6_1ff5_46d2_b8b0_9281db024326"  Port=2
  CurrMeasLoaMtgtnEna : Outport  RequirementInfo="{'linktype_rmi_doors' '0000bab3 (/E-STEER Core/SubSystem Specifications/Application Functions/SF049A Loss of Assist Manager)' '#SF049A_72' 'true' 'REQ:  SF049A_72' '' ; 'linktype_rmi_doors' '0000bab3 (/E-STEER Core/SubSystem Specifications/Application Functions/SF049A Loss of Assist Manager)' '#SF049A_73' 'true' 'REQ:  SF049A_73' '' } %GIDa_b5b5a059_d361_4603_b996_1befec25c9a9"  Port=3
  IvtrLoaMtgtnEna : Outport  RequirementInfo="{'linktype_rmi_doors' '0000bab3 (/E-STEER Core/SubSystem Specifications/Application Functions/SF049A Loss of Assist Manager)' '#SF049A_74' 'true' 'REQ:  SF049A_74' '' ; 'linktype_rmi_doors' '0000bab3 (/E-STEER Core/SubSystem Specifications/Application Functions/SF049A Loss of Assist Manager)' '#SF049A_75' 'true' 'REQ:  SF049A_75' '' } %GIDa_d6d1e458_7179_432b_aad5_f09feb5a1e87"  Port=4
  MultiMtgtnResp : Outport  RequirementInfo="{'linktype_rmi_doors' '0000bab3 (/E-STEER Core/SubSystem Specifications/Application Functions/SF049A Loss of Assist Manager)' '#SF049A_80' 'true' 'REQ:  SF049A_80' '' ; 'linktype_rmi_doors' '0000bab3 (/E-STEER Core/SubSystem Specifications/Application Functions/SF049A Loss of Assist Manager)' '#SF049A_81' 'true' 'REQ:  SF049A_81' '' ; 'linktype_rmi_doors' '0000bab3 (/E-STEER Core/SubSystem Specifications/Application Functions/SF049A Loss of Assist Manager)' '#SF049A_83' 'true' 'REQ:  SF049A_83' '' } %GIDa_9b3371e8_e728_4288_bc76_53a78185b119"  Port=5
  wires:
  HwTqResp/1 -> Relational Operator/1
  Constant/1 -> Relational Operator/2
  Relational Operator/1 -> Logical Operator1/1
  Logical Operator1/1 -> Data Store Write2/1, CntMtgtnReq/1(HwTqLoaMtgtnEna), HwTqLoaMtgtnEna/1  "HwTqLoaMtgtnEna"
  Data Store Read3/1 -> Logical Operator1/2
  MotAgResp/1 -> Relational Operator1/1
  Constant1/1 -> Relational Operator1/2
  Relational Operator1/1 -> Logical Operator2/1
  Logical Operator2/1 -> MotAgLoaMtgtnEna/1, CntMtgtnReq/2(MotAgLoaMtgtnEna), Data Store Write1/1  "MotAgLoaMtgtnEna"
  Data Store Read1/1 -> Logical Operator2/2
  CurrMeasResp/1 -> Relational Operator2/1
  Constant2/1 -> Relational Operator2/2
  Relational Operator2/1 -> Logical Operator3/1
  Logical Operator3/1 -> CurrMeasLoaMtgtnEna/1, Data Store Write3/1, CntMtgtnReq/3(CurrMeasLoaMtgtnEna)  "CurrMeasLoaMtgtnEna"
  Data Store Read2/1 -> Logical Operator3/2
  IvtrResp/1 -> Relational Operator3/1
  Constant3/1 -> Relational Operator3/2
  Relational Operator3/1 -> Logical Operator4/1
  Logical Operator4/1 -> Data Store Write4/1, CntMtgtnReq/4(IvtrLoaMtgtnEna), IvtrLoaMtgtnEna/1  "IvtrLoaMtgtnEna"
  Data Store Read4/1 -> Logical Operator4/2
  CntMtgtnReq/1(MtgtnCnt) -> If/1  "MtgtnCnt"
  If/1 -> OK_to_use/Action
  If/2 -> IllegalCombination/Action
  OK_to_use/1(Out1) -> Merge/1
  IllegalCombination/1(Out1) -> Merge/2
  Merge/1 -> MultiMtgtnResp/1

== system SF049A_LoaMgr/LoaMgr/LoaMgrPer1/Arbitrate_Responses/CopyRight2 ==
